simulink model "uio_design"  (R2022b)
settings: Solver=VariableStepAuto  StartTime=0.0  StopTime=10.0  MaxStep=0.01  RelTol=1e-3
InitFcn:
  | clear all
  | A=[0 1;-3 -2];
  | B=[0;1];
  | C=[1 0];
  | 
  | P=[-3;-3];
  | LT=acker(A',C',P);
  | L=LT';
  | 
  | E=[1;1];
  | H=E*pinv(C*E)
  | T=eye(2)-H*C
  | A1=A-H*C*A;
  | 
  | k11=4; k12=0; % we can show that one polse is always at -3 and the other pole is at -k11
  | K1=[k11;k12];
  | F=A1-K1*C
  | K2=F*H
  | K=K1+K2
settings Model: Creator=ramezani  LastModifiedBy=ramezani

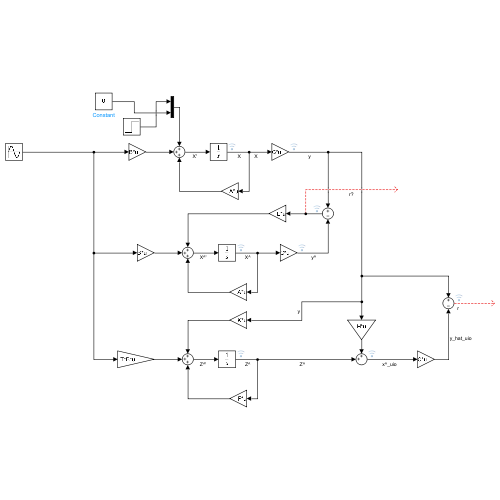
[thumbnail: Simulink's stored preview of the top-level diagram]
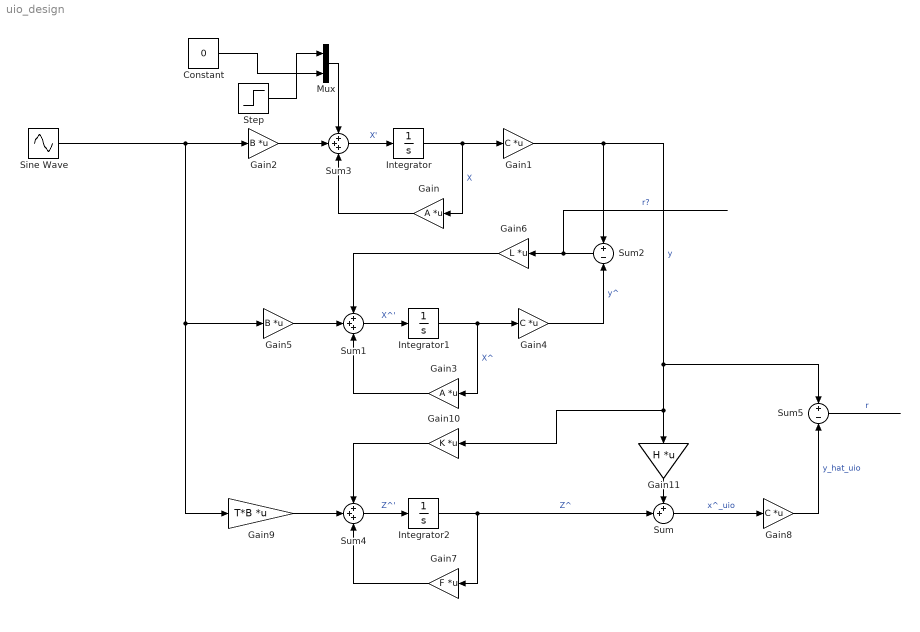
== system uio_design ==
  Constant : Constant  Value=0
  Gain : Gain  Gain=A  Multiplication=Matrix(K*u)
  Gain1 : Gain  Gain=C  Multiplication=Matrix(K*u)
  Gain10 : Gain  Gain=K  Multiplication=Matrix(K*u)
  Gain11 : Gain  Gain=H  Multiplication=Matrix(K*u)
  Gain2 : Gain  Gain=B  Multiplication=Matrix(K*u)
  Gain3 : Gain  Gain=A  Multiplication=Matrix(K*u)
  Gain4 : Gain  Gain=C  Multiplication=Matrix(K*u)
  Gain5 : Gain  Gain=B  Multiplication=Matrix(K*u)
  Gain6 : Gain  Gain=L  Multiplication=Matrix(K*u)
  Gain7 : Gain  Gain=F  Multiplication=Matrix(K*u)
  Gain8 : Gain  Gain=C  Multiplication=Matrix(K*u)
  Gain9 : Gain  Gain=T*B  Multiplication=Matrix(K*u)
  Integrator : Integrator  InitialCondition=[1;0]
  Integrator1 : Integrator
  Integrator2 : Integrator  InitialCondition=[0.5;0]
  Mux : Mux  Inputs=2
  Sine Wave : Sin  SampleTime=0
  Step : Step  Time=3  SampleTime=0
  Sum : Sum  Inputs=++|
  Sum1 : Sum  Inputs=3
  Sum2 : Sum  Inputs=+-
  Sum3 : Sum  Inputs=3
  Sum4 : Sum  Inputs=3
  Sum5 : Sum  Inputs=+-
  wires:
  Integrator/1 -> Gain1/1, Gain/1  "X"
  Gain/1 -> Sum3/3
  Sum3/1 -> Integrator/1  "X'"
  Gain2/1 -> Sum3/2
  Gain1/1 -> Sum2/1, Sum5/1, Gain10/1, Gain11/1  "y"
  Gain4/1 -> Sum2/2  "y^"
  Gain5/1 -> Sum1/2
  Sum1/1 -> Integrator1/1  "X^'"
  Gain3/1 -> Sum1/3
  Integrator1/1 -> Gain3/1, Gain4/1  "X^"
  Sum2/1 -> Gain6/1  "r?"
  Gain6/1 -> Sum1/1
  Step/1 -> Mux/1
  Gain10/1 -> Sum4/1
  Integrator2/1 -> Sum/2, Gain7/1  "Z^"
  Gain7/1 -> Sum4/3
  Sum4/1 -> Integrator2/1  "Z^'"
  Gain9/1 -> Sum4/2
  Sine Wave/1 -> Gain2/1, Gain5/1, Gain9/1
  Gain11/1 -> Sum/1
  Sum/1 -> Gain8/1  "x^_uio"
  Mux/1 -> Sum3/1
  Constant/1 -> Mux/2
  Gain8/1 -> Sum5/2  "y_hat_uio"
  Sum5/1 -> ?  "r"
